simulink model "jointSpaceTrajController_velCtrlTraj"  (Simulink 8.0)
settings: Solver=FixedStepDiscrete  StartTime=0.0  StopTime=inf  FixedStep=Ts  RelTol=1e-3
values from neighbouring files (symbols this model uses):
  qErr = 0.3    [simulinkModelinit.m]
  ROBOT_DOF = 23    [simulinkModelinit.m]
  Ts = 0.01    [simulinkModelinit.m]
undefined symbols (not defined in the file or in its folder): dqiRef, qjDes, refMask
libraries: WBCLibrary x4
settings Model: Creator=nunoguedelha  LastModifiedBy=nunoguedelha

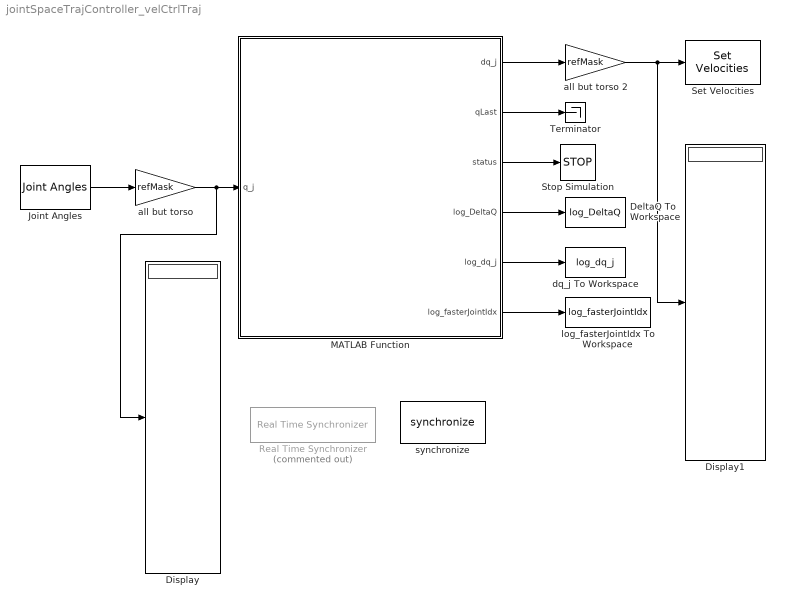
== system jointSpaceTrajController_velCtrlTraj ==
  DeltaQ To Workspace : ToWorkspace  VariableName=log_DeltaQ  SampleTime=-1  SaveFormat=Timeseries
  Display : Display
  Display1 : Display
  Joint Angles : WBCLibrary/wholeBodyStates/Joint Angles  robotName=robotName  localName=localName
  MATLAB Function : MATLAB Function  TreatAsAtomicUnit=on
  Real Time Synchronizer : WBCLibrary/Utilities/Real Time Synchronizer  Priority=-10  Commented=on  threadPeriod=Ts
  Set Velocities : WBCLibrary/wholeBodyActuators/Set Velocities  val=4  robotName=robotName  localName=localName
  Stop Simulation : Stop
  Terminator : Terminator
  all but torso : Gain  Gain=refMask
  all but torso 2 : Gain  Gain=refMask
  dq_j To Workspace : ToWorkspace  VariableName=log_dq_j  SampleTime=-1  SaveFormat=Timeseries
  log_fasterJointIdx To Workspace : ToWorkspace  VariableName=log_fasterJointIdx  SampleTime=-1  SaveFormat=Timeseries
  synchronize : WBCLibrary/Utilities/synchronize  rate=0.010  scaleFactor=1
  wires:
  Joint Angles/1 -> all but torso/1
  MATLAB Function/1(dq_j) -> all but torso 2/1
  all but torso/1 -> Display/1, MATLAB Function/1(q_j)
  all but torso 2/1 -> Display1/1, Set Velocities/1
  MATLAB Function/2(qLast) -> Terminator/1
  MATLAB Function/3(status) -> Stop Simulation/1
  MATLAB Function/4(log_DeltaQ) -> DeltaQ To Workspace/1
  MATLAB Function/5(log_dq_j) -> dq_j To Workspace/1
  MATLAB Function/6(log_fasterJointIdx) -> log_fasterJointIdx To Workspace/1

== matlab function MATLAB Function ==
  data: dq_j output double; qjDes parameter double; dqiRef parameter double; q_j input double; ROBOT_DOF parameter double; qErr parameter double; Ts parameter double; qLast output double; status output double; log_DeltaQ output double; log_dq_j output double; log_fasterJointIdx output double
function [dq_j, qLast, status, log_DeltaQ, log_dq_j, log_fasterJointIdx]  = checkStopCond(qjDes, dqiRef, q_j, ROBOT_DOF, qErr, Ts)
%#codegen

% define the maximum speed (in degrees) of the reference revolute single joint
% (single DOF). This is done manually:
% joints rotation speed is considered constant, so we only get centripete 
% acceleration . $|a_n| = \frac{v^2}{R} = R dq^2$
% => $dqiRef = \sqrt{\frac{|a_n|}{R}}$
% As a_n max should not exceed 1/10 g,
% $dqiRef = \sqrt{\frac{1}{R}} ~ sqrt(1/0.4) ~ 1.5 rad.s^{-1} = 85 degs.s^{-1}$ for $g ~
% 10m.s^{-2}$.
% Let's have a margin and define $45 deg.s^{-1}$ (signed value)
persistent fasterJointIdx;
persistent last_dq_j;
persistent last_deltaQ;
persistent stopMotionVec;
persistent state;

dq_j = zeros(ROBOT_DOF,1);

%% handle state
if isempty(state)
    state = 0;
end

% update positions relative to the destination
DeltaQ = qjDes - q_j;

% Fill static variables
if isempty(last_deltaQ)
    last_deltaQ = DeltaQ;
end

if isempty(stopMotionVec)
    stopMotionVec = ones(ROBOT_DOF,1);
end

if isempty(fasterJointIdx)
    % Select joint for which rotation will have the highest speed.
    % This shall be the high boundary speed for all joints. We shall set this
    % boundary to the maximum speed 'dqiRef' required for neglecting the angular
    % and linear acceleration to be measured by the sensors, w.r.t. the gravity
    % measurements.
    [~,idx_of_max] = max(abs(DeltaQ));
    fasterJointIdx = uint8(idx_of_max); % convert to uint8
end

if isempty(last_dq_j)
    last_dq_j = zeros(ROBOT_DOF,1);
end


if state == 0
    %% Program joint velocity for current timeslot

    % If angles are small, avoid computing dq_j, just use same velocities for
    % all joints.
    if abs(DeltaQ(fasterJointIdx))>(5*pi/180)
        dq_j = DeltaQ*(dqiRef/abs(DeltaQ(fasterJointIdx)));
        last_dq_j = dq_j;
    else
        dq_j = last_dq_j;
    end
    
    % We shall stop as soon as the joint closest to its respective end position
    % reaches the end position vicinity (d<0.1 deg) or overshoots.
    % Considering that the velocity or position tracking accuracy is not perfect, 
    % we should monitor each joint independently.
    for i = 1:ROBOT_DOF
    if abs(DeltaQ(i))<(dqiRef*10*Ts) ... % proximity
            || last_deltaQ(i)*DeltaQ(i)<0 % overshoot
        % mark respective joint for stopping
        stopMotionVec(i) = 0;
    end
    end
    
    % Stop the joints that reached destination
    dq_j = dq_j.*stopMotionVec;
    
    if any(dq_j)
        state = 0;
        last_deltaQ = DeltaQ;
    else
        % final configuration reached
        state = 1;
    end
end

% save last position
qLast = q_j;
% output state
status = state;

%log DeltaQ and dq_j
log_DeltaQ = DeltaQ;
log_dq_j = dq_j;
log_fasterJointIdx = fasterJointIdx;

% we would clear the static variables here but 'clear' is not supported
% in generated code

end
